simulink model "garmi_whole_body_ufic"  (R2022b)
settings: Solver=ode1  StartTime=0.0  StopTime=40  FixedStep=.001  RelTol=1e-3  AbsTol=1e-3
libraries: slpidlib x1, simulink x1
(part 2 of 2)

== matlab function garmi_whole_body_ufic/controller ==
  data: X_rel output; X_task input; Xd_task input; F_d input; F_pid input; tauR_ext input; tauR output; rho_z output; T_f output; T_i output; xd_tank output; Q_null input; Q input; Qdot input; Q_home input; x_tank input; Jdot_reduced input; Jreduced output
function [X_rel, tauR, rho_z, T_f, T_i, xd_tank, Jreduced] = wholeBodyUFICController(X_task, Xd_task, F_d, F_pid ,tauR_ext, Q_null, Q, Qdot, Q_home,x_tank , Jdot_reduced)

%% Define control parameters for task space
% Define gains for translation and orientation components
K_task_translation = 625; % Stiffness for translation components
K_task_orientation = 9; % Stiffness for orientation components

D_task_translation = 50; % Damping for translation components
D_task_orientation = 6; % Damping for orientation components

% Create diagonal matrices for K_task, and D_task
K_task = diag([repmat(K_task_translation, 1, 3), repmat(K_task_orientation, 1, 3), repmat(K_task_translation, 1, 3), repmat(K_task_orientation, 1, 3)]);
D_task = diag([repmat(D_task_translation, 1, 3), repmat(D_task_orientation, 1, 3), repmat(D_task_translation, 1, 3), repmat(D_task_orientation, 1, 3)]);

% Define base, right arm, and left arm gains
K_null_base = 5; % Gain for the base
D_null_base = 80; % Damping for the base

% Gains for the right arm
K_null_right_arm = 1; % Example value, adjust as needed
D_null_right_arm = 1; % Example value, adjust as needed

% Gains for the left arm
K_null_left_arm = 1; % Example value, adjust as needed (can be different from right arm if desired)
D_null_left_arm = 1; % Example value, adjust as needed (can be different from right arm if desired)

% Create diagonal matrices for K_null and D_null
K_null = diag([repmat(K_null_base, 1, 3), ...
    repmat(K_null_right_arm, 1, 7), ...
    repmat(K_null_left_arm, 1, 7)]);

D_null = diag([repmat(D_null_base, 1, 3), ...
    repmat(D_null_right_arm, 1, 7), ...
    repmat(D_null_left_arm, 1, 7)]);

%% Compute whole body task-space pose/twist and null-space vecotrs
X = [pose_arm(Q, 8, true); pose_arm(Q, 8, false)];
% Compute Whole Body Jacobian for right and left arm
Jwb_right = JacobianWholeBody(Q,8,true);
Jwb_left = JacobianWholeBody(Q,8,false);
Xdot = [Jwb_right*Qdot; Jwb_left*Qdot];

% Home positions for base and both arms
X_home = [pose_arm(Q_home, 8, true); pose_arm(Q_home, 8, false)];

% Compute task space and null space reference for the controller
X_task = X_task + X_home;
Q_null = Q_null + Q_home;
X_rel = X-X_home;

%% Compute whole body dynamics  model for the model based control.
[M, C, G] = computeDynamics(Q, Qdot);

%% Compute reduced order dynamics
% Nonholomonic contriant matrix:
A = [-sin(Q(3)), cos(Q(3)), 0, zeros(1,14)];
Adot = [-Qdot(3)*cos(Q(3)), -Qdot(3)*sin(Q(3)), 0, zeros(1,14)];

% Computations for reduced order dynamics with the nonholonimic constraint
D = [cos(Q(3)), sin(Q(3)), zeros(1,15);zeros(15,2),eye(15,15)]; % D is auxilary and arbitrary matrix to make a non-singular square constriant matrix
Ddot = [-Qdot(3)*sin(Q(3)), Qdot(3)*cos(Q(3)), zeros(1,15);zeros(15,2),zeros(15,15)];
A_D = [A;D]; % This square matrix will be used to reduce the dynamics due to its constriant.
inverse_A_D = [-sin(Q(3)), cos(Q(3)), zeros(1,15);cos(Q(3)), sin(Q(3)), zeros(1,15);zeros(15,2),eye(15,15)]; % since the D matrix is easy, we analatically inverse it
E = inverse_A_D(:,1); % if the number of the constraints are M, then the first M columns are E
F = inverse_A_D(:,2:end); % if the number of the constraints are M, then the rest of columns (N-M) are F
v = D * Qdot;  % pseudo velocities that are used as the reduced generalized coordinates of the system.
% watch this video to learn how to drive these equations:
%  https://www.youtube.com/watch?v=C1cb03fYkxk

% Compute reduced order Jacobians and Mass
Jreduced = [Jwb_right*F; Jwb_left*F];
M_reduced = F'*M*F; % Reduced mass matrix of the system.
M_reduced_inv = inv(M_reduced);
lambda = Jreduced * M_reduced_inv * Jreduced'; % auxilary variable that stores inverse of M_task.
M_task = inv(lambda);
Jr_plus_M = M_reduced_inv * Jreduced' * M_task; % compute weighted pseudo inverse
Jr_plus = Jreduced' / (Jreduced * Jreduced');

%% Map external toquese to external wrenches
J_right = JacobArm(Q,8,true);
J_left = JacobArm(Q,8,false);
J_plus_right = J_right' / (J_right * J_right');
J_plus_left = J_left' / (J_left * J_left');
F_ext = [J_plus_right' * tauR_ext(3:9);J_plus_left' * tauR_ext(10:16)];  % F_ext for right/left arm

%% UFIC Controller Design -- Tank Augmentation: Force Controller
% Select direction for force control
force_dir = [3,9];
% Compute Force Control
F_frc_ff = F_pid + F_d + K_task * (X_task - X) + F_ext;
F_frc_ff(setdiff(1:length(F_frc_ff), force_dir)) = 0;

% extract energy tank variables:
x_tf = x_tank(1);
x_ti = x_tank(2);

% Initialize variables
T_uf = 20.0;
T_lf = 0.01;
delta_Tf = 0.01;
T_ui = 20.0;
T_li = 0.01;
delta_Ti = 0.01;

% Compute the energy tank parameters for force controller
P_force = Xdot' * F_frc_ff;
T_f = 1/2 * x_tf * x_tf;
gamma_f = (P_force < 0);  % Logical condition directly assigns 1 or 0
beta_f = (T_f < T_uf);  % Logical condition directly assigns 1 or 0

if (T_f > T_lf + delta_Tf)
    alpha_f = 1;
elseif (T_lf + delta_Tf> T_f && T_f > T_lf)
    alpha_f = 1/2*(1-cos(pi*(T_f-T_lf)/(delta_Tf)));
else
    alpha_f = 0;
end

% Contact-loss stabilization
delta_frc = 0.05;
% Compute the error vector
X_tilde = X_task - X;
% Initialize rho_frc as a vector of ones (default case)
rho_frc = ones(size(X_tilde));
% Condition 1: Set rho_frc to 0 where abs(X_tilde) > 2 * delta_frc
mask1 = abs(X_tilde) >= 2 * delta_frc;
rho_frc(mask1) = 0;
% Condition 2: Apply cosine function where 0 < X_tilde <= 2 * delta_frc
mask2 = (delta_frc <= abs(X_tilde)) & (abs(X_tilde) < 2*delta_frc);  % Ensure mask1 values are excluded
rho_frc(mask2) = 0.5 * (1 + cos(pi * (X_tilde(mask2) ./ delta_frc - 1)));
% Condition 3: rho_frc remains 1 where X_tilde <= 0 (handled by initialization)
rho_z = [rho_frc(3),rho_frc(9)];

% Convert to diagonal matrix
rho_frc = diag(rho_frc);

% force control with tank augmentation:
Fp_frc_tank = rho_frc * (gamma_f + alpha_f * (1 - gamma_f)) * F_frc_ff;

%% UFIC Controller Design -- Tank Augmentation: Impedance Controller
P_impedance = Xd_task'*(Fp_frc_tank - F_ext);
T_i = 1/2*x_ti*x_ti;
gamma_i = (P_impedance > 0);  % Logical condition directly assigns 1 or 0
beta_i = (T_i < T_ui);  % Logical condition directly assigns 1 or 0

if (T_i > T_li + delta_Ti)
    alpha_i = 1;
elseif (T_li + delta_Ti> T_i && T_i > T_li)
    alpha_i = 1/2*(1-cos(pi*(T_i-T_li)/(delta_Ti)));
else
    alpha_i = 0;
end

Xd_tilde_p = (gamma_i + alpha_i * (1 - gamma_i))*Xd_task - Xdot;

% Compute energy tank dynamics:
xd_tf = -(beta_f/x_tf)*gamma_f*P_force + (alpha_f/x_tf)*(gamma_f - 1)*P_force;
xd_ti = (beta_i/x_ti)*(gamma_i*P_impedance + Xd_tilde_p'*D_task*Xd_tilde_p) + (alpha_i/x_ti)*(1-gamma_i)*P_impedance;
xd_tank = [xd_tf;xd_ti];

%% Compute force control command augmented with UFIC energy tank dynamics
a_frc_tank = -lambda * (Fp_frc_tank);
u_frc_tank = M_reduced*Jr_plus_M*(a_frc_tank);

%% Compute null space control torque command
Nr = eye(16) - Jr_plus_M*Jreduced; % compute null space.
% Compute null space torques:
tau_pid = K_null*(Q_null - Q) - D_null*(Qdot);
tau_qlim = [0 ; 0 ; 0; -JointLimitPotentialGradient(Q,true); -JointLimitPotentialGradient(Q,false)];
%tau_sa = [0 ; 0 ; 0; -SingularityAvoidanceGradient(Q,true,0.05); -SingularityAvoidanceGradient(Q,false,0.05)];
%tau_ca = [0 ; 0 ; 0; -CollisionAvoidanceGradient(Q,true); -CollisionAvoidanceGradient(Q,false)];
tau_null = tau_pid + tau_qlim; % + tau_sa + tau_ca;
u_null = M_reduced*Nr*F'*(M\(tau_null));

%% Compute task space control command -- augmented with UFIC energy tank dynamics
F_imp_tank = K_task*(X_task - X) + D_task*(Xd_tilde_p); % task space impedance wrench
a_task_tank = lambda * (F_imp_tank);
a_tauExt = -Jreduced*M_reduced_inv*tauR_ext;  % add this to u_task if you want to have disturbance rejection.
u_task = M_reduced*Jr_plus_M*(a_task_tank - Jdot_reduced*v);

%% compute whole body torque control command
u = u_task + u_null + u_frc_tank;
tauR = F'*(C*Qdot + G - M*(E*Adot + F*Ddot)*F*v) + u;

    function crossMatrix = crossOperator(vec)
        crossMatrix = [0, -vec(3), vec(2); vec(3), 0, -vec(1); -vec(2), vec(1), 0];
    end

    function T = DHmatrix(q, i)
        % Define DH parameters for each link
        l = 0.1; % Tool length
        d = [0.333, 0, 0.316, 0, 0.384, 0, 0, 0.107+l];
        a = [0, 0, 0, 0.0825, -0.0825, 0, 0.088, 0];
        alpha = [0, -pi/2, pi/2, pi/2, -pi/2, pi/2, pi/2, 0];
        q_ext = [q; 0];

        % DH Transformation matrix for the current joint
        ct = cos(q_ext(i));
        st = sin(q_ext(i));
        ca = cos(alpha(i));
        sa = sin(alpha(i));

        T = [ ct, -st, 0, a(i);
            st * ca, ct * ca, -sa, -sa * d(i);
            st * sa, ct * sa, ca, ca * d(i);
            0, 0, 0, 1];  % calculate denavit hartenberg matrix
    end

    function T_total = FK(Q, index, isRightArm)
        % Extract pose components
        x = Q(1);
        y = Q(2);
        theta = Q(3);

        % Select the correct segment of Q based on isRightArm
        if isRightArm
            q_arm = Q(4:10); % Right arm joint angles
        else
            q_arm = Q(11:17); % Left arm joint angles
        end

        % --- Parameters Definition ---
        % Base dimensions
        width = 0.75; % X-direction (width)
        height = 0.2; % Y-direction (height)
        depth = 0.75; % Z-direction (depth)

        % Wheel parameters
        wheelRadius = height / 2; % Radius of the wheels

        % Spine length along the Z-axis and offset along the Y-axis
        spineHeight = 1.05;
        spineOffset = 0.1;

        % Shoulder width along the X-axis
        shoulderWidth = 0.4;

        % Rotation matrix to compensate the installation of Franka Arms on Garmi
        % torso
        if isRightArm
            beta = pi/2.0; % Rotation about Y axis
            gamma = pi/2.0; % Rotation about Z axis
            shoulderPose = [spineOffset , -shoulderWidth/2, height+ spineHeight]; % shoulderWidth/2 m to the right
        else
            beta = pi/2.0; % Rotation about Y axis
            gamma = -pi/2.0; % Rotation about Z axis
            shoulderPose = [spineOffset  , shoulderWidth/2, height+ spineHeight]; % shoulderWidth/2 m to the left
        end

        % Transformation matrix for the base of garmi
        T_mobile_base = [cos(theta), -sin(theta), 0 , x;
            sin(theta), cos(theta) , 0 , y;
            0,          0,           1 , 0;
            0,          0,           0 ,1];
        % Transformation matrix for the shoulder pose
        Tshoulder = [1, 0, 0, shoulderPose(1);
            0, 1, 0, shoulderPose(2);
            0, 0, 1, shoulderPose(3);
            0, 0, 0, 1];

        % Transformation matrix for the Garmi wall-mount arm installation
        Ty = [cos(beta), 0, sin(beta), 0;
            0, 1, 0, 0;
            -sin(beta), 0, cos(beta), 0;
            0, 0, 0, 1];
        Tz = [cos(gamma), -sin(gamma), 0, 0;
            sin(gamma), cos(gamma), 0, 0;
            0, 0, 1, 0;
            0, 0, 0, 1];

        % Transformation of the arm_base to the universal frame
        Ti = T_mobile_base* Tshoulder * Ty * Tz;

        for arm_id = 1:index
            Ti = Ti * DHmatrix(q_arm, arm_id); % apply rotation matrix to compensate for arm configuration
        end

        T_total = Ti;
    end

    function X = pose_arm(Q, index, isRightArm)
        % init pose vector:
        X = zeros(6,1);

        % Compute the transformation matrix for the specified configuration
        T_idx = FK(Q, index, isRightArm);

        % Extract the rotation matrix from the transformation matrix
        R = T_idx(1:3, 1:3);

        % Convert the rotation matrix to an axis-angle representation
        angle = acos((trace(R) - 1) / 2);
        if angle ~= 0
            % Ensure the angle is non-zero to avoid division by zero
            axis = [R(3,2) - R(2,3); R(1,3) - R(3,1); R(2,1) - R(1,2)] / (2*sin(angle));
            % Normalize the axis to ensure it's a unit vector
            axis = axis / norm(axis);
        else
            % Handle the case of a zero angle, implying no rotation or a full rotation
            axis = [0; 0; 1]; % Default axis if no rotation is present
        end

        % return pose vector
        X(1:3)= T_idx(1:3,4);
        X(4:6) = angle * axis;
    end

    function positions = getJointsPositions(Q, isRightArm)
        positions = zeros(3, 8); % Initialize positions matrix

        for arm_id = 1:8
            T = FK(Q, arm_id, isRightArm);
            positions(:, arm_id) = T(1:3, 4); % Extract and store the position
        end
    end

    function Jacobian = JacobArm(Q, index, isRightArm)

        % Initialize the Jacobian matrix with zeros
        Jacobian = zeros(6, 7);

        % Compute FK up to the specified joint index
        T_joint_index = FK(Q, index, isRightArm);
        P_joint_index = T_joint_index(1:3, 4); % Extract the position vector of the joint at the specified index

        for arm_id = 1:index-1  % count joint positions up to one before the target joint.
            % Compute the transformation matrix up to the current joint
            Ti = FK(Q, arm_id, isRightArm);

            % Extract the joint axis of the current joint
            p_i = Ti(1:3, 4);

            % Calculate the columns of the Jacobian matrix
            z_current = Ti(1:3, 3);
            p_diff = P_joint_index - p_i;

            % Update the Jacobian matrix
            % Linear velocity part
            Jacobian(1:3, arm_id) = cross(z_current, p_diff);
            % Angular velocity part
            Jacobian(4:6, arm_id) = z_current;
        end
    end

    function Jacobian = JacobBody(Q, index, isRightArm)

        % Compute FK up to the specified joint index
        T_joint_index = FK(Q, index, isRightArm);

        % Extract the position of the joint at the specified index
        % in absolute frame relative to robot base center.
        P_joint_index = T_joint_index(1:3, 4) - [Q(1),Q(2),0]';

        % Nonholonomic matrix setup (assuming linear and angular velocity command scenario)
        nonholonomicMatrix = [1, 0, 0 ; 0, 1, 0 ; 0, 0, 0 ; 0, 0, 0 ; 0, 0, 0 ; 0, 0, 1];
        %nonholonomicMatrix = [cos(pose(3)), 0; sin(pose(3)), 0; 0, 0; 0, 0; 0, 0; 0, 1];

        % Calculate the Jacobian for the platform
        crossProdMatrix = crossOperator(P_joint_index);
        JacobianPlatform = [eye(3), -crossProdMatrix; zeros(3, 3), eye(3)];

        % Apply the nonholonomic constraints to the platform Jacobian
        Jacobian = JacobianPlatform * nonholonomicMatrix;
    end

    function J_wb = JacobianWholeBody(Q, index, isRightArm)
        J_arm = JacobArm(Q, index, isRightArm);
        J_body = JacobBody(Q, index, isRightArm);
        if isRightArm
            % Assemble the whole-body Jacobian for the right side
            J_wb = [J_body, J_arm, zeros(6, 7)];
        else
            % Assemble the whole-body Jacobian for the left side
            J_wb = [J_body, zeros(6, 7), J_arm];
        end
    end

    function jacobian = JacobArm_cg(Q, index, isRightArm)
        jacobian = zeros(6, 7); % Pre-allocate for speed
        linkCoMs = zeros(3, 7);

        % Updated CoM for each link (expressed as offsets from the link frame)
        linkCoMs = [0, -0.0256, 0.00652, -0.0472, -0.00402, 0.1263, 0.1;
            -5.844e-9, -0.323, 0.0228, 0.000919, 0.0770, -0.0410, 0.00290;
            -0.391, 0.0706, -0.0701, 0.0287, -0.376, -0.0109, 0.0272];

        T_mi = FK(Q, index, isRightArm);
        R_mi = T_mi(1:3,1:3);
        joint_position_before_mi = T_mi(1:3,4);
        r_mi_abs = joint_position_before_mi + R_mi * linkCoMs(:, index); % center of mass position of link i in global frame relative to global frame

        for joint_number = 1:index
            Ti = FK(Q,joint_number,isRightArm);
            joint_position = Ti(1:3,4);
            joint_axis = Ti(1:3,3);  % frame z axis is equivalent to the joint axis vector.

            jacobian(1:3, joint_number) = cross(joint_axis, (r_mi_abs - joint_position));
            jacobian(4:6, joint_number) = joint_axis;
        end
    end

    function Jacobian = JacobBody_cg(Q, index, isRightArm)

        % Updated CoM for each link (expressed as offsets from the link frame)
        linkCoMs = [0, -0.0256, 0.00652, -0.0472, -0.00402, 0.1263, 0.1;
            -5.844e-9, -0.323, 0.0228, 0.000919, 0.0770, -0.0410, 0.00290;
            -0.391, 0.0706, -0.0701, 0.0287, -0.376, -0.0109, 0.0272];

        % Compute FK up to the specified joint index
        T_mi = FK(Q, index, isRightArm);
        R_mi = T_mi(1:3,1:3);
        joint_position_before_cg = T_mi(1:3,4);
        r_mi_abs = joint_position_before_cg + R_mi * linkCoMs(:, index); % center of mass position of link i in global frame


        r_mi_abs_rel = r_mi_abs - [Q(1),Q(2),0]'; % center of mass position of link i relative to mobile base frame

        % Nonholonomic matrix setup (assuming linear and angular velocity command scenario)
        nonholonomicMatrix = [1, 0, 0 ; 0, 1, 0 ; 0, 0, 0 ; 0, 0, 0 ; 0, 0, 0 ; 0, 0, 1];

        % Calculate the Jacobian for the platform
        crossProdMatrix = crossOperator(r_mi_abs_rel);
        JacobianPlatform = [eye(3), -crossProdMatrix; zeros(3, 3), eye(3)];

        % Apply the nonholonomic constraints to the platform Jacobian
        Jacobian = JacobianPlatform * nonholonomicMatrix;
    end

    function J_wb = JacobianWholeBody_cg(Q, index, isRightArm)
        J_arm = JacobArm_cg(Q, index, isRightArm);
        J_body = JacobBody_cg(Q, index, isRightArm);
        if isRightArm
            % Assemble the whole-body Jacobian for the right side
            J_wb = [J_body, J_arm, zeros(6, 7)];
        else
            % Assemble the whole-body Jacobian for the left side
            J_wb = [J_body, zeros(6, 7), J_arm];
        end
    end

    function dd = calculateDistance(link1, link2) %#codegen
        coder.extrinsic('openGJK'); % Tell Simulink this is an external function
        dd = openGJK(link1, link2); % MEX function call
    end

    function coord = convertMatrix(mat)
        % Convert matrix to expected format
        numCols = size(mat, 2);
        coord = cell(1, numCols);

        for i = 1:numCols
            coord{i} = mat(1:3, i)'; % Extract the first 3 rows (assuming 3D points)
        end
    end

    function minDistances = CollisionAvoidanceDistances(Q, isRightArm)
        % Initialize minimum distances to a large value
        minDistances = ones(7,1) * inf;

        % Get joint positions for the current and opposite arm
        positions = getJointsPositions(Q, isRightArm);
        positions_other = getJointsPositions(Q, ~isRightArm);

        for i = 1:7  % avoid the first links to lower the computation load
            for j = 1:7
                % Compute link segment positions
                link = zeros(3, 3);
                link(:, 1) = positions(:, i);
                link(:, 2) = 0.5 * (positions(:, i) + positions(:, i + 1));
                link(:, 3) = positions(:, i + 1);

                link_other = zeros(3, 3);
                link_other(:, 1) = positions_other(:, j);
                link_other(:, 2) = 0.5 * (positions_other(:, j) + positions_other(:, j + 1));
                link_other(:, 3) = positions_other(:, j + 1);

                % Compute distance between the two links
                dist = calculateDistance(link, link_other);
                minDistances(i) = min(minDistances(i), dist);
            end
        end
    end

    function tau_ca = CollisionAvoidanceGradient(Q, isRightArm)
        % Internal parameters
        epsilon = 1e-6;
        Fmax = 2500;
        collisionRadius = 0.23; % Radius for collision avoidance

        tau_ca = zeros(7, 1);

        % Calculate the minimum distances of the current arm links to the other arm links
        minDistances = CollisionAvoidanceDistances(Q, isRightArm);

        % Calculate the potential at the current Q
        potential_collision_at_Q = 0;
        for i = 1:length(minDistances)
            if minDistances(i) < collisionRadius
                potential_collision_at_Q = potential_collision_at_Q - (Fmax / (collisionRadius^2) / 3) * ((minDistances(i) - collisionRadius)^3);
            end
        end

        % Determine starting index for left or right arm
        starting_index = isRightArm * 3 + ~isRightArm * 10;

        % Numerically derive the gradient
        for i = 1:7
            Q_epsilon = Q;
            Q_epsilon(i + starting_index) = Q_epsilon(i + starting_index) + epsilon;

            % Calculate minimum distances for Q_epsilon
            minDistances_epsilon = CollisionAvoidanceDistances(Q_epsilon, isRightArm);

            potential_collision_at_Q_epsilon = 0;
            for j = 1:length(minDistances_epsilon)
                if minDistances_epsilon(j) < collisionRadius
                    potential_collision_at_Q_epsilon = potential_collision_at_Q_epsilon - (Fmax / (collisionRadius^2) / 3) * ((minDistances_epsilon(j) - collisionRadius)^3);
                end
            end

            % Compute the gradient component
            tau_ca(i) = (potential_collision_at_Q_epsilon - potential_collision_at_Q) / epsilon;
        end
    end

    function tau_sa = SingularityAvoidanceGradient(Q, isRightArm, manipulability_zero)
        epsilon = 1e-6;
        k_manipulability = 200;  % Gain for the manipulability torque, avoiding high values
        tau_sa = zeros(7, 1); % Initialize gradient as a 7x1 vector

        % Compute the Jacobian (end-effector) and manipulability at Q
        J = JacobArm(Q, 8, isRightArm); % take the 6th joint position for singularity avoidance
        manipulability_at_Q = sqrt(det(J * J'));

        % Saturate k_manipulability to 50
        k_manipulability = min(k_manipulability, 200);

        % Compute the potential manipulability at Q
        if manipulability_at_Q <= manipulability_zero
            potential_manipulability_at_Q = k_manipulability * (manipulability_at_Q - manipulability_zero)^2;
        else
            potential_manipulability_at_Q = 0;
        end

        % Determine starting index for left or right arm
        starting_index = isRightArm * 3 + ~isRightArm * 10;

        % Compute gradient for each joint
        for i = 1:7
            % Perturb joint angle by epsilon
            Q_epsilon = Q;
            Q_epsilon(i + starting_index) = Q_epsilon(i + starting_index) + epsilon;

            % Compute manipulability at perturbed joint state
            J_epsilon = JacobArm(Q_epsilon, 8, isRightArm); % take the 6th joint position for singularity avoidance
            manipulability_at_Q_epsilon = sqrt(det(J_epsilon * J_epsilon'));

            % Compute the potential manipulability at Q_epsilon
            if manipulability_at_Q_epsilon <= manipulability_zero
                potential_manipulability_at_Q_epsilon = k_manipulability * (manipulability_at_Q_epsilon - manipulability_zero)^2;
            else
                potential_manipulability_at_Q_epsilon = 0;
            end

            % Compute gradient component
            tau_sa(i) = (potential_manipulability_at_Q_epsilon - potential_manipulability_at_Q) / epsilon;
        end
    end

    function tau_jlim = JointLimitPotentialGradient(Q, isRightArm)
        % Internal parameters
        delta = 0.1;
        epsilon = 1e-6;
        k_qlim = 500;

        % Hard-coded joint limits for a 7-joint robotic arm
        qmax = [2.8973; 1.7628; 2.8973; -0.0698; 2.8973; 3.7525; 2.8973];
        qmin = [-2.8973; -1.7628; -2.8973; -3.0718; -2.8973; -0.0175; -2.8973];

        tau_jlim = zeros(7, 1);
        qtilda = zeros(7, 1);

        % Determine starting index for left or right arm
        starting_index = isRightArm * 3 + ~isRightArm * 10;

        % Compute qtilda for the current Q
        for i = 1:7
            q_current = Q(i + starting_index);
            if q_current > qmax(i) - delta
                qtilda(i) = q_current - (qmax(i) - delta);
            elseif q_current < qmin(i) + delta
                qtilda(i) = q_current - (qmin(i) + delta);
            end
            % qtilda(i) remains 0 when not within delta range of limits
        end

        % Compute the potential at the current Q
        potential_jointlimit_at_Q = 0.5 * qtilda' * k_qlim * qtilda;

        % Compute gradient for each joint numerically
        for i = 1:7
            Q_epsilon = Q;
            Q_epsilon(i + starting_index) = Q_epsilon(i + starting_index) + epsilon;

            % Compute qtilda for Q_epsilon
            qtilda_epsilon = zeros(7, 1);
            for j = 1:7
                q_epsilon = Q_epsilon(j + starting_index);
                if q_epsilon > qmax(j) - delta
                    qtilda_epsilon(j) = q_epsilon - (qmax(j) - delta);
                elseif q_epsilon < qmin(j) + delta
                    qtilda_epsilon(j) = q_epsilon - (qmin(j) + delta);
                end
            end

            % Compute the potential at Q_epsilon
            potential_jointlimit_at_Q_epsilon = 0.5 * qtilda_epsilon' * k_qlim * qtilda_epsilon;

            % Compute gradient component
            tau_jlim(i) = (potential_jointlimit_at_Q_epsilon - potential_jointlimit_at_Q) / epsilon;
        end
    end

% Dynamics
    function [M, C, G] = computeDynamics(Q, Qdot)
        % Dynamic parameters
        g = [0; 0; -9.81];
        payloadMass = 0.77;

        % Updated mass for each link
        linkMasses = [4.07, 5.996, 0.570, 3.083, 3.616, 1.435, 0.453 + payloadMass];

        % Updated inertia matrices for each link, approximated and written inline
        linkInertia = zeros(3, 21);
        linkInertia(:, 1:3) = [4.47e-6, 0, 0; 0, 4.47e-6, -5.61e-10; 0, -5.61e-10, 2.00e-6]; % Link 1
        linkInertia(:, 4:6) = [0.0465, -0.00338, 0.000748; -0.00338, 0.00243, 0.00980; 0.000748, 0.00980, 0.0445]; % Link 2
        linkInertia(:, 7:9) = [0.0504, 0.00248, -0.0118; 0.00248, 0.0525, 0.00747; -0.0118, 0.00747, 0.00817]; % Link 3
        linkInertia(:, 10:12) = [0.0308, 0.00732, 0.000194; 0.00732, 0.00278, 0.00101; 0.000194, 0.00101, 0.0329]; % Link 4
        linkInertia(:, 13:15) = [0.0511, -0.000984, -0.00223; -0.000984, 0.0472, 0.00346; -0.00223, 0.00346, 0.00475]; % Link 5
        linkInertia(:, 16:18) = [0.00823, 0.00463, -0.00127; 0.00463, 0.0187, 0.00110; -0.00127, 0.00110, 0.0144]; % Link 6
        linkInertia(:, 19:21) = [0.00378, -3.27e-5, -0.000200; -3.27e-5, 0.00368, -0.000602; -0.000200, -0.000602, 0.000122]; % Link 7

        % Mass and Inertia parameters for mobile base
        baseMass = 50;
        baseInertia = 15;

        M = zeros(17, 17);
        C = zeros(17, 17);
        G = zeros(17, 1);

        % Arm dynamics computation for both arms
        for arm = 1:2 % 1 for right arm, 2 for left arm
            for arm_id = 1:7
                Tcg = FK(Q, arm_id, arm == 1);
                Rcg = Tcg(1:3, 1:3);
                Jwb_cg = JacobianWholeBody_cg(Q, arm_id, arm == 1);
                linkmass = linkMasses(arm_id);
                InertiaMatrix = reshape(linkInertia(:, 3*arm_id-2:3*arm_id), 3, 3);

                mass_link = zeros(6, 6);
                mass_link(1:3, 1:3) = linkmass * eye(3);
                mass_link(4:6, 4:6) = Rcg * InertiaMatrix * Rcg';

                Jwb_cg_v = Jwb_cg(1:3, :);

                M = M + Jwb_cg' * mass_link * Jwb_cg;
                G = G - linkmass * Jwb_cg_v' * g;
            end
            C = zeros(17, 1);
        end

        JacobBase = [eye(3),zeros(3,7),zeros(3,7)];  % jacobian of mobile base vb = JacobBase*Qdot
        % Base dynamics
        M = M + JacobBase'*diag([baseMass, baseMass, baseInertia])*JacobBase;
        G = G + zeros(17,1);
        C = C + zeros(17, 17);
    end

end

== matlab function garmi_whole_body_ufic/Momentum Observer ==
  data: Mdot input; tau_r input; Q input; Qdot input; F_ext output; tauR_ext output; moIntegral_delta output; moIntegral input
function [F_ext, tauR_ext, moIntegral_delta] = observer(Mdot, tau_r,Q,Qdot, moIntegral)

% Compute whole body dynamics  model for the model based control.
[M, C, G] = computeDynamics(Q, Qdot);

% watch this video to learn how to drive these equations:
%  https://www.youtube.com/watch?v=C1cb03fYkxk

% Nonholomonic contriant matrix:
A = [-sin(Q(3)), cos(Q(3)), 0, zeros(1,14)];
Adot = [-Qdot(3)*cos(Q(3)), -Qdot(3)*sin(Q(3)), 0, zeros(1,14)];

% Computations for reduced order dynamics considering 1DOF nonholonomic Dynamics
D = [cos(Q(3)), sin(Q(3)), zeros(1,15);zeros(15,2),eye(15,15)]; % D is auxilary and arbitrary matrix to make a non-singular square constriant matrix
Ddot = [-Qdot(3)*sin(Q(3)), Qdot(3)*cos(Q(3)), zeros(1,15);zeros(15,2),zeros(15,15)];
A_D = [A;D]; % This square matrix will be used to reduce the dynamics due to its constriant.
inverse_A_D = [-sin(Q(3)), cos(Q(3)), zeros(1,15);cos(Q(3)), sin(Q(3)), zeros(1,15);zeros(15,2),eye(15,15)]; % since the D matrix is easy, we analatically inverse it
E = inverse_A_D(:,1); % if the number of the constraints are M, then the first M columns are E
F = inverse_A_D(:,2:end); % if the number of the constraints are M, then the rest of columns (N-M) are F
v = D * Qdot;  % pseudo velocities that are used as the reduced generalized coordinates of the system.

% Momentum Observer
KI = 500;
M_reduced = F'*M*F; % Reduced mass matrix of the system.
Momentum = M_reduced * v;
residual = KI * (Momentum - moIntegral);
moIntegral_delta = tau_r + F'*(Mdot - (E*Adot + F*Ddot)'*M')*F*v -F'*G + residual;
tauR_ext = residual;

% Map external toquese to external forces
J_right = JacobArm(Q,8,true);
J_left = JacobArm(Q,8,false);
J_plus_right = J_right' / (J_right * J_right');
J_plus_left = J_left' / (J_left * J_left');
F_ext = [J_plus_right' * tauR_ext(3:9);J_plus_left' * tauR_ext(10:16)];  % F_ext for right/left arm

    function crossMatrix = crossOperator(vec)
        crossMatrix = [0, -vec(3), vec(2); vec(3), 0, -vec(1); -vec(2), vec(1), 0];
    end

    function T = DHmatrix(q, i)
        % Define DH parameters for each link
        l = 0.1; % Tool length
        d = [0.333, 0, 0.316, 0, 0.384, 0, 0, 0.107+l];
        a = [0, 0, 0, 0.0825, -0.0825, 0, 0.088, 0];
        alpha = [0, -pi/2, pi/2, pi/2, -pi/2, pi/2, pi/2, 0];
        q_ext = [q; 0];

        % DH Transformation matrix for the current joint
        ct = cos(q_ext(i));
        st = sin(q_ext(i));
        ca = cos(alpha(i));
        sa = sin(alpha(i));

        T = [ ct, -st, 0, a(i);
            st * ca, ct * ca, -sa, -sa * d(i);
            st * sa, ct * sa, ca, ca * d(i);
            0, 0, 0, 1];  % calculate denavit hartenberg matrix
    end

    function T_total = FK(Q, index, isRightArm)
        % Extract pose components
        x = Q(1);
        y = Q(2);
        theta = Q(3);

        % Select the correct segment of Q based on isRightArm
        if isRightArm
            q_arm = Q(4:10); % Right arm joint angles
        else
            q_arm = Q(11:17); % Left arm joint angles
        end

        % --- Parameters Definition ---
        % Base dimensions
        width = 0.75; % X-direction (width)
        height = 0.2; % Y-direction (height)
        depth = 0.75; % Z-direction (depth)

        % Wheel parameters
        wheelRadius = height / 2; % Radius of the wheels

        % Spine length along the Z-axis and offset along the Y-axis
        spineHeight = 1.05;
        spineOffset = 0.1;

        % Shoulder width along the X-axis
        shoulderWidth = 0.4;

        % Rotation matrix to compensate the installation of Franka Arms on Garmi
        % torso
        if isRightArm
            beta = pi/2.0; % Rotation about Y axis
            gamma = pi/2.0; % Rotation about Z axis
            shoulderPose = [spineOffset , -shoulderWidth/2, height+ spineHeight]; % shoulderWidth/2 m to the right
        else
            beta = pi/2.0; % Rotation about Y axis
            gamma = -pi/2.0; % Rotation about Z axis
            shoulderPose = [spineOffset  , shoulderWidth/2, height+ spineHeight]; % shoulderWidth/2 m to the left
        end

        % Transformation matrix for the base of garmi
        T_mobile_base = [cos(theta), -sin(theta), 0 , x;
            sin(theta), cos(theta) , 0 , y;
            0,          0,           1 , 0;
            0,          0,           0 ,1];
        % Transformation matrix for the shoulder pose
        Tshoulder = [1, 0, 0, shoulderPose(1);
            0, 1, 0, shoulderPose(2);
            0, 0, 1, shoulderPose(3);
            0, 0, 0, 1];

        % Transformation matrix for the Garmi wall-mount arm installation
        Ty = [cos(beta), 0, sin(beta), 0;
            0, 1, 0, 0;
            -sin(beta), 0, cos(beta), 0;
            0, 0, 0, 1];
        Tz = [cos(gamma), -sin(gamma), 0, 0;
            sin(gamma), cos(gamma), 0, 0;
            0, 0, 1, 0;
            0, 0, 0, 1];

        % Transformation of the arm_base to the universal frame
        Ti = T_mobile_base* Tshoulder * Ty * Tz;

        for arm_id = 1:index
            Ti = Ti * DHmatrix(q_arm, arm_id); % apply rotation matrix to compensate for arm configuration
        end

        T_total = Ti;
    end

    function X = pose_arm(Q, index, isRightArm)
        % init pose vector:
        X = zeros(6,1);

        % Compute the transformation matrix for the specified configuration
        T_idx = FK(Q, index, isRightArm);

        % Extract the rotation matrix from the transformation matrix
        R = T_idx(1:3, 1:3);

        % Convert the rotation matrix to an axis-angle representation
        angle = acos((trace(R) - 1) / 2);
        if angle ~= 0
            % Ensure the angle is non-zero to avoid division by zero
            axis = [R(3,2) - R(2,3); R(1,3) - R(3,1); R(2,1) - R(1,2)] / (2*sin(angle));
            % Normalize the axis to ensure it's a unit vector
            axis = axis / norm(axis);
        else
            % Handle the case of a zero angle, implying no rotation or a full rotation
            axis = [0; 0; 1]; % Default axis if no rotation is present
        end

        % return pose vector
        X(1:3)= T_idx(1:3,4);
        X(4:6) = angle * axis;
    end

    function positions = getJointsPositions(Q, isRightArm)
        positions = zeros(3, 8); % Initialize positions matrix

        for arm_id = 1:8
            T = FK(Q, arm_id, isRightArm);
            positions(:, arm_id) = T(1:3, 4); % Extract and store the position
        end
    end

    function Jacobian = JacobArm(Q, index, isRightArm)

        % Initialize the Jacobian matrix with zeros
        Jacobian = zeros(6, 7);

        % Compute FK up to the specified joint index
        T_joint_index = FK(Q, index, isRightArm);
        P_joint_index = T_joint_index(1:3, 4); % Extract the position vector of the joint at the specified index

        for arm_id = 1:index-1  % count joint positions up to one before the target joint.
            % Compute the transformation matrix up to the current joint
            Ti = FK(Q, arm_id, isRightArm);

            % Extract the joint axis of the current joint
            P_i = Ti(1:3, 4);

            % Calculate the columns of the Jacobian matrix
            z_current = Ti(1:3, 3);
            p_diff = P_joint_index - P_i;

            % Update the Jacobian matrix
            % Linear velocity part
            Jacobian(1:3, arm_id) = cross(z_current, p_diff);
            % Angular velocity part
            Jacobian(4:6, arm_id) = z_current;
        end
    end

    function Jacobian = JacobBody(Q, index, isRightArm)

        % Compute FK up to the specified joint index
        T_joint_index = FK(Q, index, isRightArm);

        % Extract the position of the joint at the specified index
        % in absolute frame relative to robot base center.
        P_joint_index = T_joint_index(1:3, 4) - [Q(1),Q(2),0]';

        % Nonholonomic matrix setup (assuming linear and angular velocity command scenario)
        nonholonomicMatrix = [1, 0, 0 ; 0, 1, 0 ; 0, 0, 0 ; 0, 0, 0 ; 0, 0, 0 ; 0, 0, 1];
        %nonholonomicMatrix = [cos(pose(3)), 0; sin(pose(3)), 0; 0, 0; 0, 0; 0, 0; 0, 1];

        % Calculate the Jacobian for the platform
        crossProdMatrix = crossOperator(P_joint_index);
        JacobianPlatform = [eye(3), -crossProdMatrix; zeros(3, 3), eye(3)];

        % Apply the nonholonomic constraints to the platform Jacobian
        Jacobian = JacobianPlatform * nonholonomicMatrix;
    end

    function J_wb = JacobianWholeBody(Q, index, isRightArm)
        J_arm = JacobArm(Q, index, isRightArm);
        J_body = JacobBody(Q, index, isRightArm);
        if isRightArm
            % Assemble the whole-body Jacobian for the right side
            J_wb = [J_body, J_arm, zeros(6, 7)];
        else
            % Assemble the whole-body Jacobian for the left side
            J_wb = [J_body, zeros(6, 7), J_arm];
        end
    end

    function jacobian = JacobArm_cg(Q, index, isRightArm)
        jacobian = zeros(6, 7); % Pre-allocate for speed
        linkCoMs = zeros(3, 7);

        % Updated CoM for each link (expressed as offsets from the link frame)
        linkCoMs = [0, -0.0256, 0.00652, -0.0472, -0.00402, 0.1263, 0.1;
            -5.844e-9, -0.323, 0.0228, 0.000919, 0.0770, -0.0410, 0.00290;
            -0.391, 0.0706, -0.0701, 0.0287, -0.376, -0.0109, 0.0272];

        T_mi = FK(Q, index, isRightArm);
        R_mi = T_mi(1:3,1:3);
        joint_position_before_mi = T_mi(1:3,4);
        r_mi_abs = joint_position_before_mi + R_mi * linkCoMs(:, index); % center of mass position of link i in global frame relative to global frame

        for joint_number = 1:index
            Ti = FK(Q,joint_number,isRightArm);
            joint_position = Ti(1:3,4);
            joint_axis = Ti(1:3,3);  % frame z axis is equivalent to the joint axis vector.

            jacobian(1:3, joint_number) = cross(joint_axis, (r_mi_abs - joint_position));
            jacobian(4:6, joint_number) = joint_axis;
        end
    end

    function Jacobian = JacobBody_cg(Q, index, isRightArm)

        % Updated CoM for each link (expressed as offsets from the link frame)
        linkCoMs = [0, -0.0256, 0.00652, -0.0472, -0.00402, 0.1263, 0.1;
            -5.844e-9, -0.323, 0.0228, 0.000919, 0.0770, -0.0410, 0.00290;
            -0.391, 0.0706, -0.0701, 0.0287, -0.376, -0.0109, 0.0272];

        % Compute FK up to the specified joint index
        T_mi = FK(Q, index, isRightArm);
        R_mi = T_mi(1:3,1:3);
        joint_position_before_cg = T_mi(1:3,4);
        r_mi_abs = joint_position_before_cg + R_mi * linkCoMs(:, index); % center of mass position of link i in global frame


        r_mi_abs_rel = r_mi_abs - [Q(1),Q(2),0]'; % center of mass position of link i relative to mobile base frame

        % Nonholonomic matrix setup (assuming linear and angular velocity command scenario)
        nonholonomicMatrix = [1, 0, 0 ; 0, 1, 0 ; 0, 0, 0 ; 0, 0, 0 ; 0, 0, 0 ; 0, 0, 1];

        % Calculate the Jacobian for the platform
        crossProdMatrix = crossOperator(r_mi_abs_rel);
        JacobianPlatform = [eye(3), -crossProdMatrix; zeros(3, 3), eye(3)];

        % Apply the nonholonomic constraints to the platform Jacobian
        Jacobian = JacobianPlatform * nonholonomicMatrix;
    end

    function J_wb = JacobianWholeBody_cg(Q, index, isRightArm)
        J_arm = JacobArm_cg(Q, index, isRightArm);
        J_body = JacobBody_cg(Q, index, isRightArm);
        if isRightArm
            % Assemble the whole-body Jacobian for the right side
            J_wb = [J_body, J_arm, zeros(6, 7)];
        else
            % Assemble the whole-body Jacobian for the left side
            J_wb = [J_body, zeros(6, 7), J_arm];
        end
    end

% Dynamics
    function [M, C, G] = computeDynamics(Q, Qdot)
        % Dynamic parameters
        g = [0; 0; -9.81];
        payloadMass = 0.77;

        % Updated mass for each link
        linkMasses = [4.07, 5.996, 0.570, 3.083, 3.616, 1.435, 0.453 + payloadMass];

        % Updated inertia matrices for each link, approximated and written inline
        linkInertia = zeros(3, 21);
        linkInertia(:, 1:3) = [4.47e-6, 0, 0; 0, 4.47e-6, -5.61e-10; 0, -5.61e-10, 2.00e-6]; % Link 1
        linkInertia(:, 4:6) = [0.0465, -0.00338, 0.000748; -0.00338, 0.00243, 0.00980; 0.000748, 0.00980, 0.0445]; % Link 2
        linkInertia(:, 7:9) = [0.0504, 0.00248, -0.0118; 0.00248, 0.0525, 0.00747; -0.0118, 0.00747, 0.00817]; % Link 3
        linkInertia(:, 10:12) = [0.0308, 0.00732, 0.000194; 0.00732, 0.00278, 0.00101; 0.000194, 0.00101, 0.0329]; % Link 4
        linkInertia(:, 13:15) = [0.0511, -0.000984, -0.00223; -0.000984, 0.0472, 0.00346; -0.00223, 0.00346, 0.00475]; % Link 5
        linkInertia(:, 16:18) = [0.00823, 0.00463, -0.00127; 0.00463, 0.0187, 0.00110; -0.00127, 0.00110, 0.0144]; % Link 6
        linkInertia(:, 19:21) = [0.00378, -3.27e-5, -0.000200; -3.27e-5, 0.00368, -0.000602; -0.000200, -0.000602, 0.000122]; % Link 7


        % Mass and Inertia parameters for mobile base
        baseMass = 50;
        baseInertia = 15;

        M = zeros(17, 17);
        C = zeros(17, 17);
        G = zeros(17, 1);

        % Arm dynamics computation for both arms
        for arm = 1:2 % 1 for right arm, 2 for left arm
            for arm_id = 1:7
                Tcg = FK(Q, arm_id, arm == 1);
                Rcg = Tcg(1:3, 1:3);
                Jwb_cg = JacobianWholeBody_cg(Q, arm_id, arm == 1);
                linkmass = linkMasses(arm_id);
                InertiaMatrix = reshape(linkInertia(:, 3*arm_id-2:3*arm_id), 3, 3);

                mass_link = zeros(6, 6);
                mass_link(1:3, 1:3) = linkmass * eye(3);
                mass_link(4:6, 4:6) = Rcg * InertiaMatrix * Rcg';

                Jwb_cg_v = Jwb_cg(1:3, :);

                M = M + Jwb_cg' * mass_link * Jwb_cg;
                G = G - linkmass * Jwb_cg_v' * g;
            end
            C = zeros(17, 1);
        end

        JacobBase = [eye(3),zeros(3,7),zeros(3,7)];  % jacobian of mobile base vb = JacobBase*Qdot
        % Base dynamics
        M = M + JacobBase'*diag([baseMass, baseMass, baseInertia])*JacobBase;
        G = G + zeros(17,1);
        C = C + zeros(17, 17);
    end
end
